simulink model "lab2_part1"  (R2022a)
settings: Solver=VariableStepAuto  StartTime=0.0  StopTime=30  RelTol=10e-10  AbsTol=10e-10
settings Model: Creator=yuans  LastModifiedBy=yuans

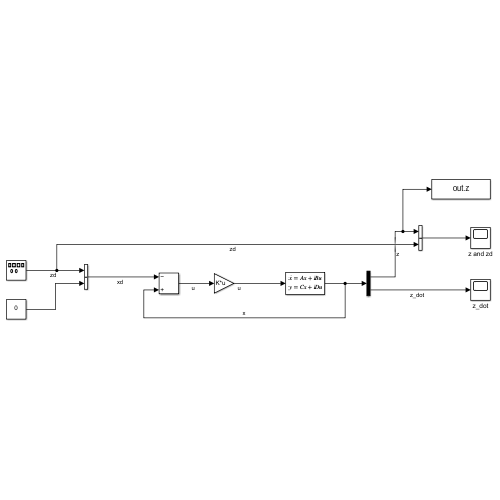
[thumbnail: Simulink's stored preview of the top-level diagram]
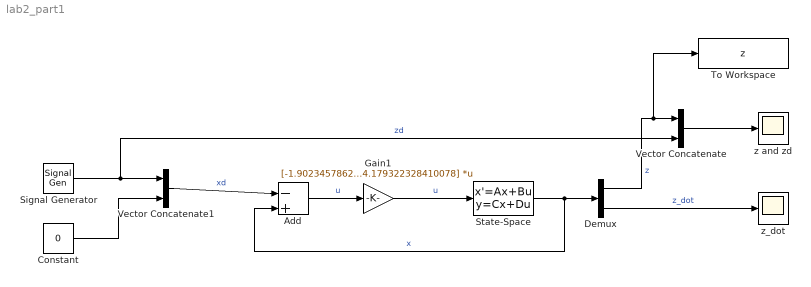
== system lab2_part1 ==
  Add : Sum  Inputs=-|+
  Constant : Constant  Value=0
  Demux : Demux  Outputs=2
  Gain1 : Gain  Gain=[-1.902345786272806 4.179322328410078]  Multiplication=Matrix(K*u)
  Signal Generator : SignalGenerator  WaveForm=square  Amplitude=0.03  Frequency=0.1  VectorParams1D=off
  State-Space : StateSpace  A=[0 1;0 -12.787723785166239]  B=[0;2.102667153818049]  C=[1 0;0 1]  D=[0;0]  InitialCondition=0  ParameterTunability=Unconstrained
  To Workspace : ToWorkspace  VariableName=z  SaveFormat=Timeseries  SampleTime=-1
  Vector Concatenate : Concatenate
  Vector Concatenate1 : Concatenate
  z and zd : Scope
  z_dot : Scope
  wires:
  Add/1 -> Gain1/1  "u"
  State-Space/1 -> Add/2, Demux/1  "x"
  Vector Concatenate1/1 -> Add/1  "xd"
  Signal Generator/1 -> Vector Concatenate/2, Vector Concatenate1/1  "zd"
  Constant/1 -> Vector Concatenate1/2
  Vector Concatenate/1 -> z and zd/1
  Demux/2 -> z_dot/1  "z_dot"
  Gain1/1 -> State-Space/1  "u"
  Demux/1 -> To Workspace/1, Vector Concatenate/1  "z"
